simulink model "tire"  (R2024b)
settings: Solver=VariableStepAuto  StartTime=0.0  StopTime=10  RelTol=1e-3
libraries: simulink x2
settings Model: Creator=Pain  LastModifiedBy=Pain

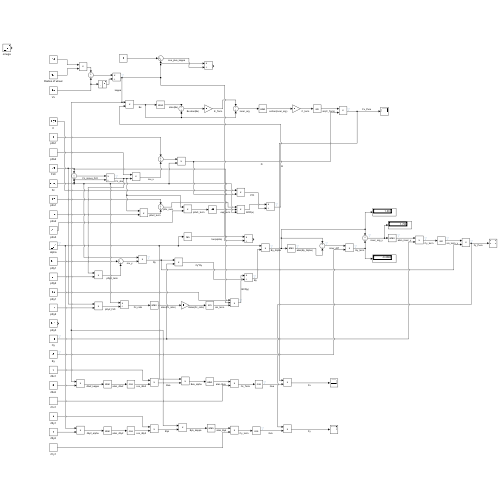
[thumbnail: Simulink's stored preview of the top-level diagram]
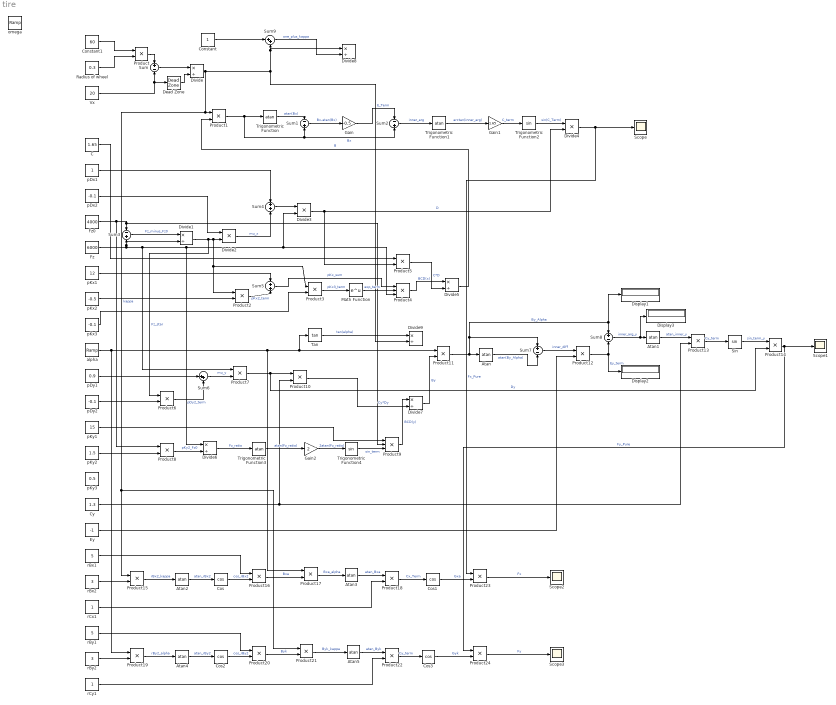
== system tire ==
  Atan{,1..5} (6 alike) : Trigonometry  Operator=atan
  C : Constant  Value=1.65
  Constant : Constant
  Constant1 : Constant  Value=60
  Cos{,1..3} (4 alike) : Trigonometry  Operator=cos
  Cy : Constant  Value=1.3
  Dead Zone : DeadZone
  Display1 : Display
  Display2 : Display
  Display3 : Display
  Divide{,1,5..9} (7 alike) : Product  Inputs=*/
  Divide2 : Product  Inputs=**
  Divide3 : Product  Inputs=**
  Divide4 : Product  Inputs=**
  Ey : Constant  Value=-1
  Fz : Constant  Value=6000
  Fz0 : Constant  Value=4000
  Gain : Gain  Gain=-0.5
  Gain1 : Gain  Gain=1.65
  Gain2 : Gain  Gain=2
  Math Function : Math
  Product{,1..3,5..8,10..24} (23 alike) : Product
  Product4 : Product  Inputs=3
  Product9 : Product  Inputs=3
  Radius of wheel : Constant  Value=0.3
  Scope{,1..3} (4 alike) : Scope
  Sin : Trigonometry
  Sum : Sum  Inputs=+-
  Sum1 : Sum  Inputs=-+
  Sum2 : Sum  Inputs=-+
  Sum3 : Sum  Inputs=-+
  Sum4 : Sum
  Sum5 : Sum  Inputs=+|+
  Sum6 : Sum  Inputs=|++
  Sum7 : Sum  Inputs=+-
  Sum8 : Sum  Inputs=+-
  Sum9 : Sum  Inputs=|++
  Tan : Trigonometry  Operator=tan
  Trigonometric Function : Trigonometry  Operator=atan
  Trigonometric Function1 : Trigonometry  Operator=atan
  Trigonometric Function2 : Trigonometry
  Trigonometric Function3 : Trigonometry  Operator=atan
  Trigonometric Function4 : Trigonometry
  Vx : Constant  Value=20
  alpha : simulink/Sources/Ramp  slope=0.03  start=0  InitialOutput=-0.15
  omega : simulink/Sources/Ramp  slope=20  start=0  InitialOutput=0
  pDx1 : Constant
  pDx2 : Constant  Value=-0.1
  pDy1 : Constant  Value=0.9
  pDy2 : Constant  Value=-0.1
  pKx1 : Constant  Value=12
  pKx2 : Constant  Value=-0.5
  pKx3 : Constant  Value=-0.1
  pKy1 : Constant  Value=15
  pKy2 : Constant  Value=1.5
  pKy3 : Constant  Value=0.5
  rBx1 : Constant  Value=5
  rBx2 : Constant  Value=3
  rBy1 : Constant  Value=5
  rBy2 : Constant  Value=3
  rCx1 : Constant
  rCy1 : Constant
  wires:
  Constant1/1 -> Product/1
  Radius of wheel/1 -> Product/2
  Product/1 -> Sum/1
  Vx/1 -> Dead Zone/1, Sum/2
  Sum/1 -> Divide/1
  Dead Zone/1 -> Divide/2
  Divide/1 -> Divide8/1, Sum9/2, Divide9/2, Product21/1, Product15/1, Product1/1  "kappa"
  Product1/1 -> Sum2/2, Sum1/2, Trigonometric Function/1  "Bx"
  Trigonometric Function/1 -> Sum1/1  "atan(Bx)"
  Sum1/1 -> Gain/1  "Bx-atan(Bx)"
  Gain/1 -> Sum2/1  "E_Term"
  Sum2/1 -> Trigonometric Function1/1  "inner_arg"
  Trigonometric Function1/1 -> Gain1/1  "arctan(inner_arg)"
  Gain1/1 -> Trigonometric Function2/1  "C_term"
  Trigonometric Function2/1 -> Divide4/1  "sin(C_Term)"
  Divide4/1 -> Product23/1, Scope/1  "Fx_Pure"
  Fz0/1 -> Product8/1, Product9/2, Sum3/1
  Fz/1 -> Divide6/1, Product4/3, Divide3/2, Product7/1, Divide1/2, Sum3/2
  Sum3/1 -> Divide1/1  "Fz_minus_Fz0"
  Divide1/1 -> Product6/1, Product3/1, Product2/1, Divide2/2  "Fz_star"
  pDx2/1 -> Divide2/1
  Divide2/1 -> Sum4/2  "mu_x"
  pDx1/1 -> Sum4/1
  Sum4/1 -> Divide3/1
  Divide3/1 -> Product5/2, Divide4/2  "D"
  pKx2/1 -> Product2/2
  Product2/1 -> Sum5/2  "pKx2_term"
  pKx1/1 -> Sum5/1
  Sum5/1 -> Product4/1  "pKx_sum"
  pKx3/1 -> Product3/2
  Product3/1 -> Math Function/1  "pKx3_term"
  Math Function/1 -> Product4/2  "exp_term"
  C/1 -> Product5/1
  Product5/1 -> Divide5/2  "C*D"
  Divide5/1 -> Product1/2  "B"
  Product4/1 -> Divide5/1  "BCD(x)"
  pDy2/1 -> Product6/2
  pDy1/1 -> Sum6/1
  Product6/1 -> Sum6/2  "pDy2_term"
  Sum6/1 -> Product7/2  "mu_y"
  pKy2/1 -> Product8/2
  Product8/1 -> Divide6/2  "pKy2_Fz0"
  Divide6/1 -> Trigonometric Function3/1  "Fz_ratio"
  Trigonometric Function3/1 -> Gain2/1  "atan(Fz_ratio)"
  Gain2/1 -> Trigonometric Function4/1  "2atan(Fz_ratio)"
  pKy1/1 -> Product9/1
  Product7/1 -> Product14/2, Product10/1  "Dy"
  Cy/1 -> Product13/2, Product10/2
  Product10/1 -> Divide7/2  "Cy*Dy"
  Product9/1 -> Divide7/1  "BCD(y)"
  alpha/1 -> Product19/1, Product17/1, Tan/1, Product11/1
  Divide7/1 -> Product11/2  "By"
  Product11/1 -> Sum8/1, Display1/1, Sum7/1, Atan/1  "By_Alpha"
  Atan/1 -> Sum7/2  "atan(By_Alpha)"
  Sum7/1 -> Product12/1  "inner_diff"
  Ey/1 -> Product12/2
  Product12/1 -> Sum8/2, Display2/1  "Ey_term"
  Sum8/1 -> Display3/1, Atan1/1  "inner_arg_y"
  Atan1/1 -> Product13/1  "atan_inner_y"
  Product13/1 -> Sin/1  "Cy_term"
  Sin/1 -> Product14/1  "sin_term_y"
  Product14/1 -> Product24/1, Scope1/1  "Fy_Pure"
  Trigonometric Function4/1 -> Product9/3  "sin_term"
  Constant/1 -> Sum9/1
  Sum9/1 -> Divide8/2  "one_plus_kappa"
  Tan/1 -> Divide9/1  "tan(alpha)"
  rBx2/1 -> Product15/2
  Product15/1 -> Atan2/1  "rBx2_kappa"
  Atan2/1 -> Cos/1  "atan_rBx2"
  Cos/1 -> Product16/2  "cos_rBx2"
  rBx1/1 -> Product16/1
  Product16/1 -> Product17/2  "Bxa"
  Product17/1 -> Atan3/1  "Bxa_alpha"
  Atan3/1 -> Product18/1  "atan_Bxa"
  rCx1/1 -> Product18/2
  Product18/1 -> Cos1/1  "Cx_Term"
  rBy2/1 -> Product19/2
  Product19/1 -> Atan4/1  "rBy2_alpha"
  Atan4/1 -> Cos2/1  "atan_rBy2"
  Cos2/1 -> Product20/2  "cos_rBy2"
  rBy1/1 -> Product20/1
  Product20/1 -> Product21/2  "Byk"
  Product21/1 -> Atan5/1  "Byk_kappa"
  Atan5/1 -> Product22/1  "atan_Byk"
  rCy1/1 -> Product22/2
  Product22/1 -> Cos3/1  "Cy_term"
  Cos1/1 -> Product23/2  "Gxa"
  Cos3/1 -> Product24/2  "Gyk"
  Product24/1 -> Scope3/1  "Fy"
  Product23/1 -> Scope2/1  "Fx"
